simulink model "schema_di_controllo_progetto_esame"  (R2023b)
settings: Solver=VariableStepAuto  StartTime=0.0  StopTime=700  RelTol=1e-3
values from neighbouring files (symbols this model uses):
  C = [1 0]    [progetto_esame.m]
  u_e = T_diff/k * log(1/(1 - (m*gg*r_2)/(K_max * r_1 * (l - r_1 * x_1e))) - 1) + T_avg    [progetto_esame.m]
  WW = 1    [progetto_esame.m]
  x_1e = pi/3    (= 1.0471975512)    [progetto_esame.m]
  x_2e = 0    [progetto_esame.m]
libraries: cstblocks x3
settings Model: SimulationMode=accelerator  Creator=evang  LastModifiedBy=evang

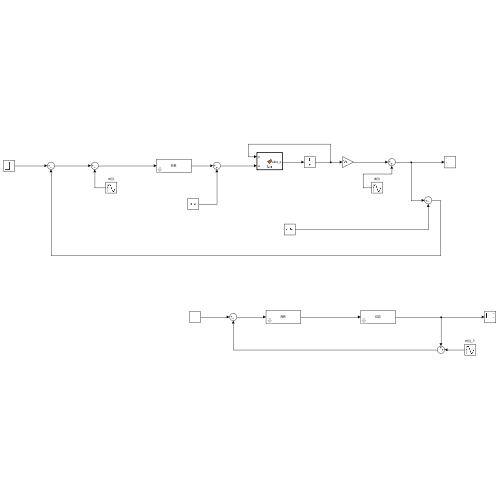
[thumbnail: Simulink's stored preview of the top-level diagram]
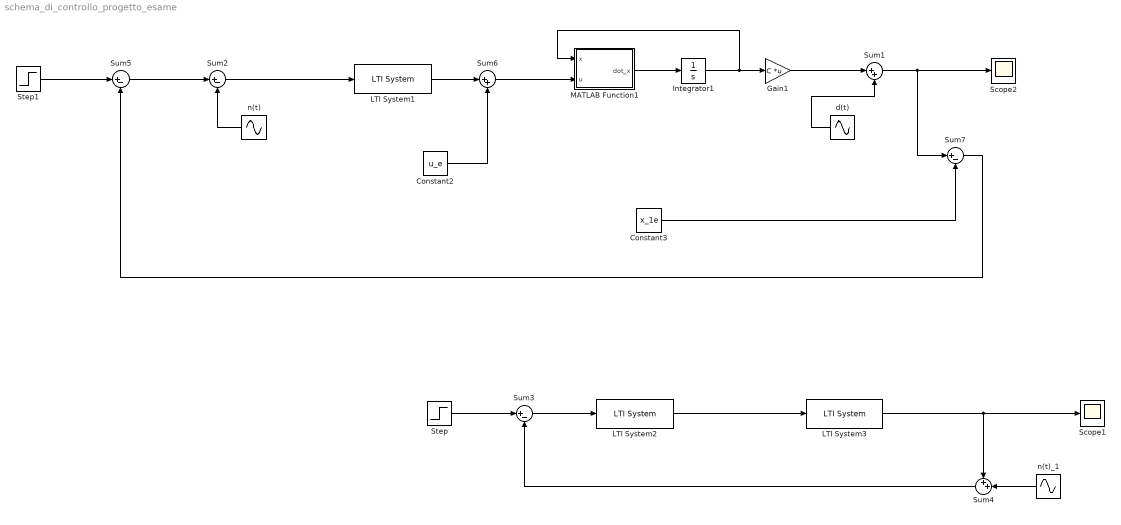
== system schema_di_controllo_progetto_esame ==
  Constant2 : Constant  Value=u_e
  Constant3 : Constant  Value=x_1e
  Gain1 : Gain  Gain=C  Multiplication=Matrix(K*u)
  Integrator1 : Integrator  InitialCondition=[x_1e;x_2e]
  LTI System1 : cstblocks/LTI System  sys=RR  IC=[]  PadeOrder=0
  LTI System2 : cstblocks/LTI System  sys=RR  IC=[]  PadeOrder=0
  LTI System3 : cstblocks/LTI System  sys=GG  IC=[]  PadeOrder=0
  MATLAB Function1 : MATLAB Function  TreatAsAtomicUnit=on
  Scope1 : Scope
  Scope2 : Scope
  Step : Step  Time=0  After=WW  SampleTime=0
  Step1 : Step  Time=0  After=WW  SampleTime=0
  Sum1 : Sum  Inputs=|++
  Sum{2..3,5,7} (4 alike) : Sum  Inputs=|+-
  Sum4 : Sum  Inputs=++|
  Sum6 : Sum  Inputs=|++
  d(t) : Sin  Amplitude=0.01  Frequency=0.01  SampleTime=0
  n(t) : Sin  Amplitude=0.01  Frequency=10000  SampleTime=0
  n(t)_1 : Sin  Amplitude=0.01  Frequency=1000  SampleTime=0
  wires:
  LTI System3/1 -> Sum4/1, Scope1/1
  Step/1 -> Sum3/1
  Sum3/1 -> LTI System2/1
  n(t)_1/1 -> Sum4/2
  Sum4/1 -> Sum3/2
  Constant3/1 -> Sum7/2
  Sum7/1 -> Sum5/2
  LTI System1/1 -> Sum6/1
  Constant2/1 -> Sum6/2
  MATLAB Function1/1(dot_x) -> Integrator1/1
  Integrator1/1 -> MATLAB Function1/1(x), Gain1/1
  Sum6/1 -> MATLAB Function1/2(u)
  Step1/1 -> Sum5/1
  LTI System2/1 -> LTI System3/1
  Gain1/1 -> Sum1/1
  Sum1/1 -> Sum7/1, Scope2/1
  d(t)/1 -> Sum1/2
  Sum5/1 -> Sum2/1
  Sum2/1 -> LTI System1/1
  n(t)/1 -> Sum2/2

== matlab function schema_di_controllo_progetto_esame/MATLAB Function1 ==
  data: x input; u input; dot_x output
function dot_x = fcn(x,u)

m = 0.04;       % [kg] massa
beta = 0.08;    % coefficiente
r_2 = 0.045;    % [m] raggio esterno puleggia
r_1 = 0.0045;   % [m] raggio interno puleggia
l = 1;          % 
J = 0.962;      % [kg m^2] momento di inerzia
K_max = 4000;   % 
k = 6.2;        % coefficiente
T_avg = 70;     % temperatura media
T_diff = 20;    % differenza di temperatura
gg = 9.81;      % [kg/ms^2] costante di gravitazione universale


dot_x = zeros(2,1);

dot_x(1) = x(2);

dot_x(2) = (K_max*(1-1/(1+exp(k*(u-T_avg)/T_diff)))*(l-r_1*x(1))*r_1 - (m*gg + beta * r_2 * x(2) *r_2))/J
